simulink model "ros_teleop"  (R2021a)
settings: Solver=FixedStepDiscrete  StartTime=0.0  StopTime=inf  FixedStep=0.05  RelTol=1e-3
model workspace (MAT data in the model file):
  SL_ROS_VariableLengthArrays_MaxSizes.CommonInfo.ArrayTruncateAction = 'EmitWarning'
  SL_ROS_VariableLengthArrays_MaxSizes.MsgTypeMap = containers.Map
  SL_ROS_VariableLengthArrays_MaxSizes.MsgTypeMap.serialization.keys = {'sensor_msgs/Image'}
  SL_ROS_VariableLengthArrays_MaxSizes.MsgTypeMap.serialization.values{1}(1).PropertyName = 'Data'
  SL_ROS_VariableLengthArrays_MaxSizes.MsgTypeMap.serialization.values{1}(1).DataType = 'uint8'
  SL_ROS_VariableLengthArrays_MaxSizes.MsgTypeMap.serialization.values{1}(1).MaxLength = 2764800
  SL_ROS_VariableLengthArrays_MaxSizes.MsgTypeMap.serialization.values{1}(2).PropertyName = 'Encoding'
  SL_ROS_VariableLengthArrays_MaxSizes.MsgTypeMap.serialization.values{1}(2).DataType = 'uint8'
  SL_ROS_VariableLengthArrays_MaxSizes.MsgTypeMap.serialization.values{1}(2).MaxLength = 921600
  SL_ROS_VariableLengthArrays_MaxSizes.MsgTypeMap.serialization.uniformity = 0
  SL_ROS_VariableLengthArrays_MaxSizes.MsgTypeMap.serialization.keyType = 'char'
  SL_ROS_VariableLengthArrays_MaxSizes.MsgTypeMap.serialization.valueType = 'any'
libraries: robotlib x4, dspvision x1, visionsinks x1
settings Model: EnablePacing=on  Creator=The MathWorks, Inc.  LastModifiedBy=tkikawad
settings SolverCC: AlgebraicLoopSolver=TrustRegion
settings DataIOCC: ReturnWorkspaceOutputs=off
settings OptimizationCC: LifeSpan=inf  MaxStackSize=64  EfficientTunableParamExpr=on
settings DebuggingCC: ParameterPrecisionLossMsg=none  ParameterTunabilityLossMsg=error  PregeneratedLibrarySubsystemCodeDiagnostic=none  SFExecutionAtInitializationDiag=none  SFMachineParentedDataDiag=warning  ArithmeticOperatorsInVariantConditions=warning
settings HardwareCC: ProdBitPerLong=64  ProdHWDeviceType=Intel->x86-64 (Linux 64)
settings SFSimCC: SimUseLocalCustomCode=off  MATLABDynamicMemAlloc=off  CustomCodeUndefinedFunction=UseInterfaceOnly  SimTargetLang=C++
settings RTWCC: SystemTargetFile=ert.tlc  HardwareBoard=Robot Operating System (ROS)  TLCOptions="-aInlineSetEventsForThisBaseRateFcn=TLC_FALSE -aSuppressMultiTaskScheduler=TLC_FALSE  -aRateBasedStepFcn=0"  TemplateMakefile=ert_default_tmf  GenerateReport=on  RTWUseLocalCustomCode=off  Toolchain=Catkin  IncludeHyperlinkInReport=on  LaunchReport=on  TargetLang=C++  GenerateTraceInfo=on  GenerateTraceReport=on  GenerateTraceReportSl=on  GenerateTraceReportSf=on  GenerateTraceReportEml=on  GenerateWebview=on
settings CodeAppCC: ForceParamTrailComments=on  IgnoreCustomStorageClasses=off  OperatorAnnotations=on  SimulinkDataObjDesc=on  SFDataObjDesc=on  MATLABFcnDesc=on  InsertBlockDesc=on  StateflowObjectComments=on  MATLABSourceComments=on
settings ERTTargetCC: TargetLangStandard=C99 (ISO)  MultiwordLength=2048  SupportVariableSizeSignals=on
settings ConfigComp: CovMetricSettings=dsw  CovSaveCumulativeToWorkspaceVar=on  CovSaveSingleToWorkspaceVar=on  CovExternalEMLEnable=off
settings SimscapeCC: SimscapeNormalizeSystem=off

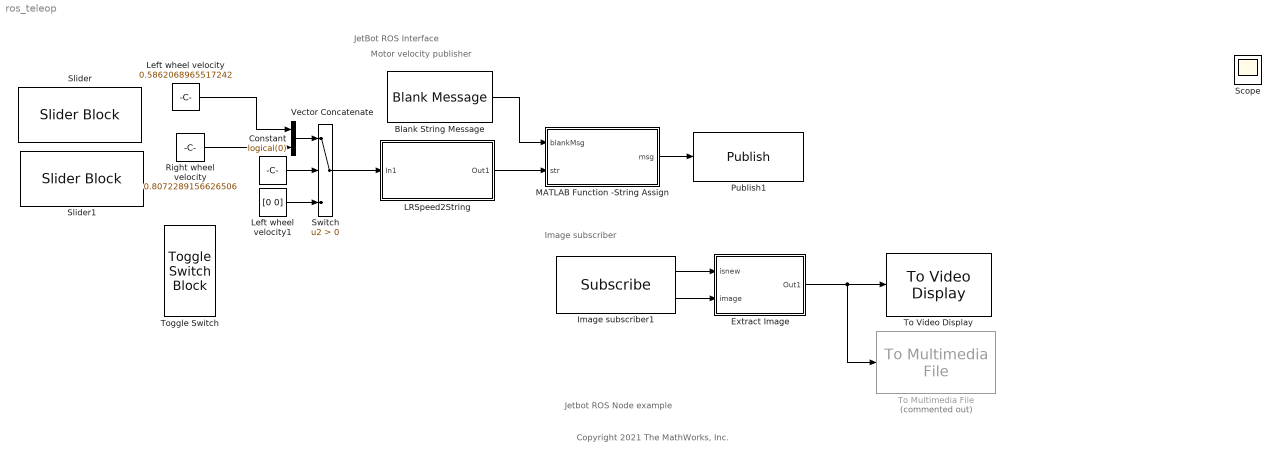
== system ros_teleop ==
  note: Image subscriber
  note: Motor velocity publisher
  note: JetBot ROS Interface
  note: Jetbot ROS Node example
  note: Copyright 2021 The MathWorks, Inc.
  Blank String Message : robotlib/Blank Message  messageClass=Message  entityType=std_msgs/String  messageType=std_msgs/String  SampleTime=inf  legacyBusStruct=off
  Constant : Constant  Value=logical(0)
  Extract Image : Subsystem
  Image subscriber1 : robotlib/Subscribe  topicSource=Select from ROS network  topic=/image_raw  messageType=sensor_msgs/Image  SampleTime=0.1  legacyBusStruct=off  messageQueueLength=1
      link override SourceBlock: ROSTopic=/jetbot_camera/raw  ROSMessageType=sensor_msgs/Image  SLBusName=SL_Bus_ballTracker_sensor_msgs_Image  ModelName=ballTracker  BlockId=Sub_ballTracker_201
  LRSpeed2String : Subsystem
  Left wheel velocity : Constant  Value=0.5862068965517242  SampleTime=0.1
  Left wheel velocity1 : Constant  Value=[0 0]  SampleTime=0.1
  MATLAB Function -String Assign : MATLAB Function  TreatAsAtomicUnit=on
  Publish1 : robotlib/Publish  topicSource=Select from ROS network  topic=/jetbot_motors/cmd_raw  messageType=std_msgs/String  legacyBusStruct=off  messageQueueLength=1
  Right wheel velocity : Constant  Value=0.8072289156626506  SampleTime=0.1
  Slider : SliderBlock  ScaleMin=-1  ScaleMax=1
  Slider1 : SliderBlock  ScaleMin=-1  ScaleMax=1
  Switch : Switch  Criteria=u2 > Threshold
  To Multimedia File : dspvision/To Multimedia File  Commented=on  outputFilename=trainVideo_sl.avi  streamSelection=Video only  videoCompressor=None (uncompressed)  audioCompressor=None (uncompressed)  imagePorts=One multidimensional signal  fileType=AVI  audioDatatype=Determine from input data type  fourcc=RGB  videoQuality=75  mj2000CompFactor=10
  To Video Display : visionsinks/To Video Display  windowSizeMode=Normal  openAtMdlStart=on  fullScreen=off  videoWindowX=-329  videoWindowY=257  saveWindowSize=off  videoWindowWidth=321  videoWindowHeight=190  inputColorFormat=RGB  inputType=Obsolete  imagePorts=One multidimensional signal  OutputDevice=On-screen video monitor  dataOrg=Column-major  isWindowOpen=off
  Toggle Switch : ToggleSwitchBlock
      settings: Values={{'Off', 'On'}, [0 1]}
  Vector Concatenate : Concatenate
  Scope : Scope
  wires:
  Right wheel velocity/1 -> Vector Concatenate/2
  Left wheel velocity/1 -> Vector Concatenate/1
  Vector Concatenate/1 -> Switch/1
  Extract Image/1(Out1) -> To Multimedia File/1, To Video Display/1
  Constant/1 -> Switch/2
  Left wheel velocity1/1 -> Switch/3
  Switch/1 -> LRSpeed2String/1(In1)
  LRSpeed2String/1(Out1) -> MATLAB Function -String Assign/2(str)
  MATLAB Function -String Assign/1(msg) -> Publish1/1
  Image subscriber1/2 -> Extract Image/2(image)
  Image subscriber1/1 -> Extract Image/1(isnew)
  Blank String Message/1 -> MATLAB Function -String Assign/1(blankMsg)

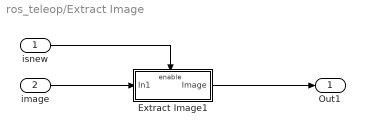
== system ros_teleop/Extract Image ==
  isnew : Inport
  image : Inport  Port=2
  Extract Image1 : Subsystem
  Out1 : Outport
  wires:
  Extract Image1/1(Image) -> Out1/1
  image/1 -> Extract Image1/1(In1)
  isnew/1 -> Extract Image1/Enable

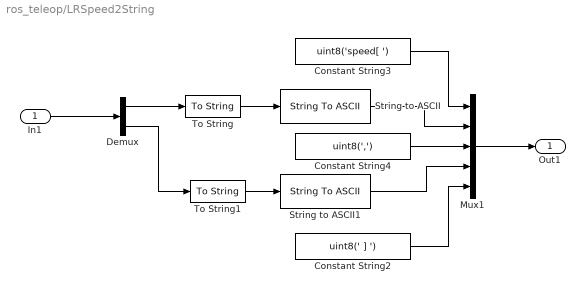
== system ros_teleop/LRSpeed2String ==
  In1 : Inport
  Constant String2 : Constant  Value=uint8(' ] ')
  Constant String3 : Constant  Value=uint8('speed[ ')
  Constant String4 : Constant  Value=uint8(',')
  Demux : Demux  Outputs=2
  Mux1 : Mux  Inputs=5
  String to ASCII : StringToASCII  OutputVectorSize=4
  String to ASCII1 : StringToASCII  OutputVectorSize=4
  To String : ToString
  To String1 : ToString
  Out1 : Outport  VectorParamsAs1DForOutWhenUnconnected=off
  wires:
  String to ASCII/1 -> Mux1/2
  Demux/1 -> To String/1
  Constant String4/1 -> Mux1/3
  Constant String3/1 -> Mux1/1
  Demux/2 -> To String1/1
  To String1/1 -> String to ASCII1/1
  To String/1 -> String to ASCII/1
  Constant String2/1 -> Mux1/5
  String to ASCII1/1 -> Mux1/4
  Mux1/1 -> Out1/1
  In1/1 -> Demux/1

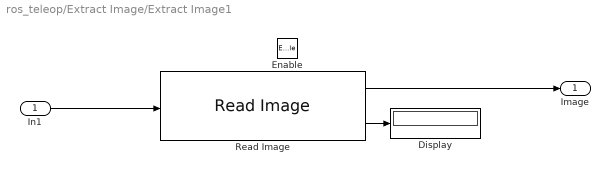
== system ros_teleop/Extract Image/Extract Image1 ==
  In1 : Inport
  Enable : EnablePort
  Display : Display
  Read Image : robotlib/Read Image  MaximumImageSize=[180, 320]  ImageEncoding=bgr8  ShowAlphaOutput=off  ShowErrorCodeOutput=on  VariableSizeOutputs=off
      settings: SourceProductBaseCode=RR
  Image : Outport  VectorParamsAs1DForOutWhenUnconnected=off
  wires:
  Read Image/1 -> Image/1
  In1/1 -> Read Image/1
  Read Image/2 -> Display/1

== matlab function ros_teleop/MATLAB Function -String Assign ==
  data: blankMsg input Bus: SL_Bus_ros_teleop_std_msgs_String; msg output Bus: SL_Bus_ros_teleop_std_msgs_String; str input
function msg = assignStringInput(blankMsg, str)
% assignStringInput - Assign a string in a ROS message to specified input string
%
% MSG = assignStringInput(blankMsg, STR) assigns the input string, STR, to
%  a string field in the ROS message, blankMsg, and outputs the updated
%  ROS message.
%
%  Inputs
%    blankMsg: A bus for a 'std_msgs/String' message. This is 
%        used to initialize the output.
%    str: An array of uint8 that will be assigned to the 'Data' field
%        in blankMsg. The entire array is assumed to be a valid sequence of
%        character ASCII values.
% 
%  Outputs:
%    msg: A bus for a 'std_msgs/String' message, with the 'Data'
%        field set to a string.

%   Copyright 2015 The MathWorks, Inc.
%#codegen

% Note: The datatype of 'msg' has been explicitly set to the appropriate 
% Simulink bus type ("Bus: SL_Bus_robotROSMessageUsageExample_std_msgs_String"). 
%
% If the model name is changed, the datatype needs to be changed as well:
%   1) Click "Edit Data" in the Editor toolstrip to open "Ports and Data Manager"
%   2) Select "msg". From the "Type" dropdown, select "--- Refresh data types ---"
%   3) Set datatype to "Bus: SL_Bus_<modelname>_std_msgs_String"
    
msg = blankMsg;

% msg (std_msgs/String) consists of
%           Data : array of type uint8
%   Data_SL_Info : struct with fields CurrentLength, ReceivedLength
strLength = length(str);
msg.Data(1:strLength) = str;
msg.Data_SL_Info.CurrentLength = uint32(strLength);
